simulink model "Nov15"  (Simulink 7.9)
settings: Solver=ode1  StartTime=0.0  StopTime=inf  FixedStep=0.002  RelTol=1e-3
undefined symbols (not defined in the file): HIL
libraries: quarc_library x5, simulink x2
settings Model: Creator=ald5  LastModifiedBy=Philip  SimulationMode=external  ExtModeTrigDuration=10000
settings SolverCC: PositivePriorityOrder=on
settings DebuggingCC: FcnCallInpInsideContextMsg=Use local settings  StrictBusMsg=Warning
settings RTWCC: SystemTargetFile=quarc_windows.tlc  TemplateMakefile=quarc_default_tmf  Description=QuaRC Win32 Target  ProcessScript=quarc_windows_make_rtw_hook
settings STFCustomTargetCC: TargetPreCompLibLocation=C:\DOCUME~1\ALLUSE~1\APPLIC~1\QuaRC\lib\2009b\windows\release  CodeReplacementLibrary=ANSI_C  GeneratePreprocessorConditionals=Disable all  SystemTargetFile=quarc_windows.tlc
settings GRTTargetCC: TargetPreCompLibLocation=C:\DOCUME~1\ALLUSE~1\APPLIC~1\QuaRC\lib\2009b\windows\release  ParMdlRefBuildCompliant=off  CompOptLevelCompliant=off  ConcurrentExecutionCompliant=off  CombineOutputUpdateFcns=off  MatFileLogging=off  GRTInterface=on  ExtMode=on  ExtModeMexFile=quarc_comm

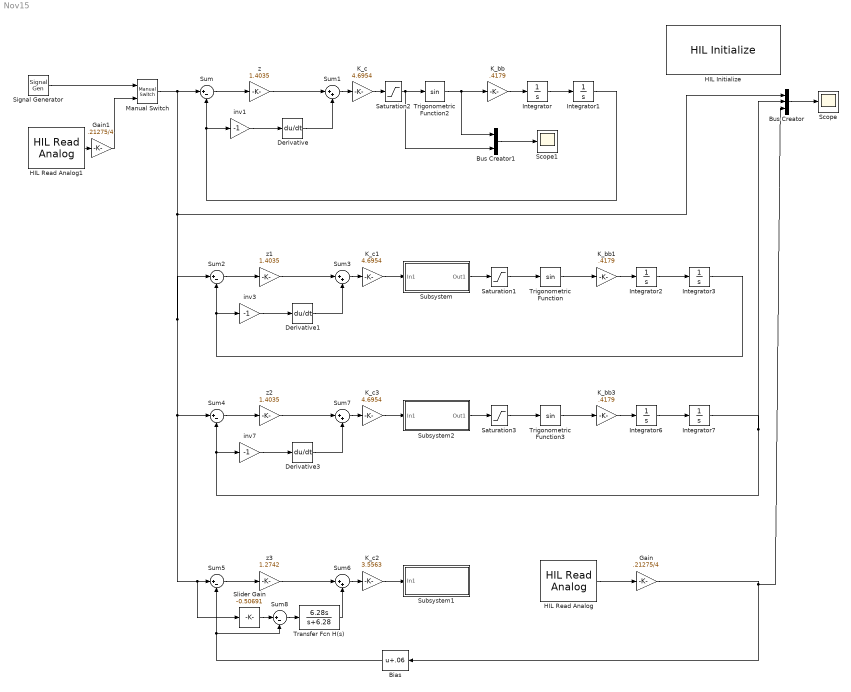
== system Nov15 ==
  Bias : Bias  Bias=.06
  Bus Creator : BusCreator  Inputs=3
  Bus Creator1 : BusCreator  Inputs=2
  Derivative : Derivative
  Derivative1 : Derivative
  Derivative3 : Derivative
  Gain : Gain  Gain=.21275/4
  Gain1 : Gain  Gain=.21275/4
  HIL Initialize : quarc_library/Data Acquisition/Generic/Configuration/HIL Initialize  object_name=HIL-1  board_type=q4  board_number=0  exclusive=off  active=off  hardware_clocks=[0:1]  clock_modes=[0 0]  set_clock_params_at_start=on  set_clock_params_at_switch_in=off  analog_input_channels=[0:3]  analog_input_maximums=10  analog_input_minimums=-10  set_analog_input_params_at_start=off  set_analog_input_params_at_switch_in=off  analog_output_channels=[0:3]  analog_output_maximums=[10]  analog_output_minimums=[-10]  initial_analog_outputs=[0]  final_analog_outputs=[0]  watchdog_analog_outputs=0  set_analog_output_params_at_start=on  set_analog_output_params_at_switch_in=off  set_analog_outputs_at_start=on  set_analog_outputs_at_switch_in=off  set_analog_outputs_at_terminate=on  set_analog_outputs_at_switch_out=off  set_analog_outputs_on_watchdog=off  digital_input_channels=[]  digital_output_channels=[]  digital_output_configuration=[]  initial_digital_outputs=[1]  final_digital_outputs=[1]  watchdog_digital_outputs=[2]  set_digital_output_params_at_start=off  set_digital_output_params_at_switch_in=off  set_digital_outputs_at_start=on  set_digital_outputs_at_switch_in=off  set_digital_outputs_at_terminate=on  set_digital_outputs_at_switch_out=off  set_digital_outputs_on_watchdog=off  encoder_channels=[0:3]  quadrature=[4]  encoder_filter_frequency=(1/60e-9)/1  initial_encoder_counts=[0]  set_encoder_params_at_start=on  set_encoder_params_at_switch_in=off  set_encoder_counts_at_start=on  set_encoder_counts_at_switch_in=off  pwm_channels=[]  pwm_modes=[0]  pwm_frequency=(1/60e-9)/1024  pwm_configuration=[]  pwm_alignment=[]  pwm_polarity=[]  pwm_leading_deadband=[]  pwm_trailing_deadband=[]  initial_pwm_outputs=[0]  final_pwm_outputs=[0]  watchdog_pwm_outputs=[]  set_pwm_params_at_start=on  set_pwm_params_at_switch_in=off  set_pwm_outputs_at_start=on  set_pwm_outputs_at_switch_in=off  set_pwm_outputs_at_terminate=on  set_pwm_outputs_at_switch_out=off  set_pwm_outputs_on_watchdog=off  other_output_channels=[]  initial_other_outputs=[]  final_other_outputs=[]  watchdog_other_outputs=[]  set_other_outputs_at_start=off  set_other_outputs_at_switch_in=off  set_other_outputs_at_terminate=off  set_other_outputs_at_switch_out=off  set_other_outputs_on_watchdog=off
  HIL Read Analog : quarc_library/Data Acquisition/Generic/Immediate I//O/HIL Read Analog  object_name=HIL-1  channels=[2]  sample_time=qc_get_step_size  active=on  vector_output=off
  HIL Read Analog1 : quarc_library/Data Acquisition/Generic/Immediate I//O/HIL Read Analog  object_name=HIL-1  channels=[3]  sample_time=qc_get_step_size  active=on  vector_output=off
  Integrator{,1..3,6..7} (6 alike) : Integrator
  K_bb : Gain  Gain=.4179
  K_bb1 : Gain  Gain=.4179
  K_bb3 : Gain  Gain=.4179
  K_c : Gain  Gain=4.6954
  K_c1 : Gain  Gain=4.6954
  K_c2 : Gain  Gain=3.5563
  K_c3 : Gain  Gain=4.6954
  Manual Switch : simulink/Signal Routing/Manual Switch  sw=1  action=0  varsize=off
  Saturation1 : Saturate  UpperLimit=1  LowerLimit=-1
  Saturation2 : Saturate  UpperLimit=1  LowerLimit=-1
  Saturation3 : Saturate  UpperLimit=1  LowerLimit=-1
  Scope : Scope
      settings: YMin=-0.15  YMax=0.25
  Scope1 : Scope
      settings: YMin=-0.1  YMax=0.25
  Signal Generator : SignalGenerator  WaveForm=square  Amplitude=.1  Frequency=.2  Units=rad/sec
  Slider Gain : simulink/Math Operations/Slider Gain  low=-1  gain=-0.50691  high=0
  Subsystem : Subsystem
  Subsystem1 : Subsystem
  Subsystem2 : Subsystem
  Sum{,2,4..5,8} (5 alike) : Sum  Inputs=|+-
  Sum{1,3,6..7} (4 alike) : Sum  Inputs=|++
  Transfer Fcn H(s) : TransferFcn  Numerator=[6.28 0]  Denominator=[1 6.28]
  Trigonometric Function : Trigonometry
  Trigonometric Function2 : Trigonometry
  Trigonometric Function3 : Trigonometry
  inv1 : Gain  Gain=-1
  inv3 : Gain  Gain=-1
  inv7 : Gain  Gain=-1
  z : Gain  Gain=1.4035
  z1 : Gain  Gain=1.4035
  z2 : Gain  Gain=1.4035
  z3 : Gain  Gain=1.2742
  wires:
  Manual Switch/1 -> Sum/1, Sum2/1, Sum4/1, Sum5/1, Slider Gain/1, Bus Creator/1
  Bus Creator/1 -> Scope/1
  K_bb1/1 -> Integrator2/1
  Integrator2/1 -> Integrator3/1
  z1/1 -> Sum3/1
  Sum2/1 -> z1/1
  inv3/1 -> Derivative1/1
  Derivative1/1 -> Sum3/2
  Sum3/1 -> K_c1/1
  Integrator3/1 -> Sum2/2, inv3/1
  K_c1/1 -> Subsystem/1(In1)
  K_bb3/1 -> Integrator6/1
  Integrator6/1 -> Integrator7/1
  z2/1 -> Sum7/1
  Sum4/1 -> z2/1
  inv7/1 -> Derivative3/1
  Derivative3/1 -> Sum7/2
  Sum7/1 -> K_c3/1
  Integrator7/1 -> Sum4/2, inv7/1, Bus Creator/2
  K_c3/1 -> Subsystem2/1(In1)
  Subsystem2/1(Out1) -> Saturation3/1
  Saturation3/1 -> Trigonometric Function3/1
  Trigonometric Function3/1 -> K_bb3/1
  Subsystem/1(Out1) -> Saturation1/1
  Saturation1/1 -> Trigonometric Function/1
  Trigonometric Function/1 -> K_bb1/1
  z3/1 -> Sum6/1
  Sum5/1 -> z3/1
  Slider Gain/1 -> Sum8/1
  Sum8/1 -> Transfer Fcn H(s)/1
  Sum6/1 -> K_c2/1
  Gain/1 -> Bus Creator/3, Bias/1
  K_c2/1 -> Subsystem1/1(In1)
  K_bb/1 -> Integrator/1
  Integrator/1 -> Integrator1/1
  z/1 -> Sum1/1
  Sum/1 -> z/1
  inv1/1 -> Derivative/1
  Derivative/1 -> Sum1/2
  Sum1/1 -> K_c/1
  Integrator1/1 -> Sum/2, inv1/1
  Trigonometric Function2/1 -> K_bb/1, Bus Creator1/1
  Bus Creator1/1 -> Scope1/1
  K_c/1 -> Saturation2/1
  Saturation2/1 -> Trigonometric Function2/1, Bus Creator1/2
  Transfer Fcn H(s)/1 -> Sum6/2
  HIL Read Analog/1 -> Gain/1
  Bias/1 -> Sum5/2, Sum8/2
  Signal Generator/1 -> Manual Switch/1
  HIL Read Analog1/1 -> Gain1/1
  Gain1/1 -> Manual Switch/2

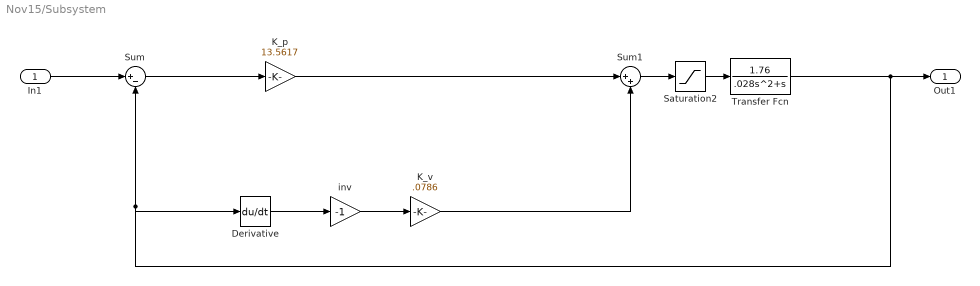
== system Nov15/Subsystem ==
  In1 : Inport
  Derivative : Derivative
  K_p : Gain  Gain=13.5617
  K_v : Gain  Gain=.0786
  Saturation2 : Saturate  UpperLimit=10  LowerLimit=-10
  Sum : Sum  Inputs=|+-
  Sum1 : Sum  Inputs=|++
  Transfer Fcn : TransferFcn  Numerator=[1.76]  Denominator=[.028 1 0]
  inv : Gain  Gain=-1
  Out1 : Outport
  wires:
  Sum/1 -> K_p/1
  K_p/1 -> Sum1/1
  Transfer Fcn/1 -> Sum/2, Derivative/1, Out1/1
  Sum1/1 -> Saturation2/1
  inv/1 -> K_v/1
  Derivative/1 -> inv/1
  K_v/1 -> Sum1/2
  Saturation2/1 -> Transfer Fcn/1
  In1/1 -> Sum/1

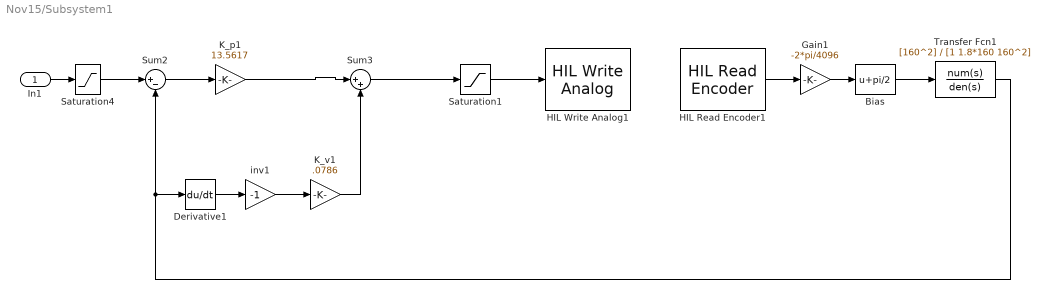
== system Nov15/Subsystem1 ==
  In1 : Inport
  Bias : Bias  Bias=pi/2
  Derivative1 : Derivative
  Gain1 : Gain  Gain=-2*pi/4096
  HIL Read Encoder1 : quarc_library/Data Acquisition/Generic/Immediate I//O/HIL Read Encoder  object_name=HIL-1  channels=0  sample_time=qc_get_step_size  active=on  vector_output=off  data_type_mode=Inherit via back propagation  data_type=double
  HIL Write Analog1 : quarc_library/Data Acquisition/Generic/Immediate I//O/HIL Write Analog  object_name=HIL-1  channels=0  sample_time=-1  active=off  vector_input=off
  K_p1 : Gain  Gain=13.5617
  K_v1 : Gain  Gain=.0786
  Saturation1 : Saturate  UpperLimit=10  LowerLimit=-10
  Saturation4 : Saturate  UpperLimit=1  LowerLimit=-1
  Sum2 : Sum  Inputs=|+-
  Sum3 : Sum  Inputs=|++
  Transfer Fcn1 : TransferFcn  Numerator=[160^2]  Denominator=[1 1.8*160 160^2]
  inv1 : Gain  Gain=-1
  wires:
  Sum2/1 -> K_p1/1
  Sum3/1 -> Saturation1/1
  Derivative1/1 -> inv1/1
  Saturation1/1 -> HIL Write Analog1/1
  Gain1/1 -> Bias/1
  inv1/1 -> K_v1/1
  K_p1/1 -> Sum3/1
  In1/1 -> Saturation4/1
  K_v1/1 -> Sum3/2
  Transfer Fcn1/1 -> Sum2/2, Derivative1/1
  Saturation4/1 -> Sum2/1
  HIL Read Encoder1/1 -> Gain1/1
  Bias/1 -> Transfer Fcn1/1

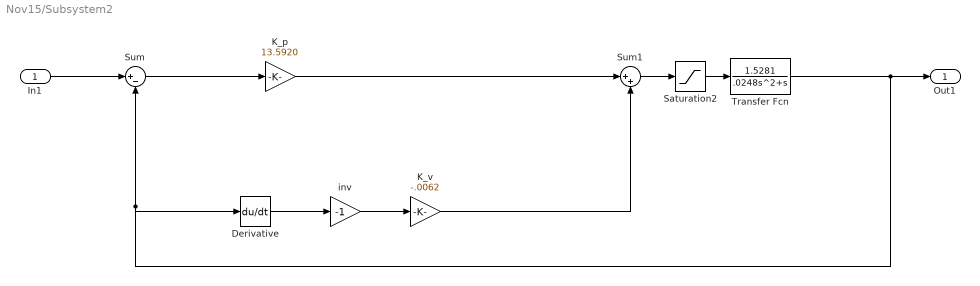
== system Nov15/Subsystem2 ==
  In1 : Inport
  Derivative : Derivative
  K_p : Gain  Gain=13.5920
  K_v : Gain  Gain=-.0062
  Saturation2 : Saturate  UpperLimit=10  LowerLimit=-10
  Sum : Sum  Inputs=|+-
  Sum1 : Sum  Inputs=|++
  Transfer Fcn : TransferFcn  Numerator=[1.5281]  Denominator=[.0248 1 0]
  inv : Gain  Gain=-1
  Out1 : Outport
  wires:
  Sum/1 -> K_p/1
  K_p/1 -> Sum1/1
  Transfer Fcn/1 -> Sum/2, Derivative/1, Out1/1
  Sum1/1 -> Saturation2/1
  inv/1 -> K_v/1
  Derivative/1 -> inv/1
  K_v/1 -> Sum1/2
  Saturation2/1 -> Transfer Fcn/1
  In1/1 -> Sum/1
